simulink model "ampelkreuzungV1.1"  (R2024b)
settings: Solver=FixedStepAuto  StartTime=0.0  StopTime=300  FixedStep=1  RelTol=1e-3
model workspace (MATLAB code in the model file):
  | function [autos_l1, autos_rg1, autos_2l, autos_2rg, autos_3l, autos_3rg, autos_4, fehler] = generateCars(Auslastung)
  |     if (auslastung == 1)
  |         autos_l1 = round(randn());
  |         autos_rg1 = round(randn());
  |         autos_2l = round(randn());
  |         autos_2rg = round(randn());
  |         autos_3l = round(randn());
  |         autos_3rg = round(randn());
  |         autos_4 = round(randn());
  |     else
  |         fehler = 1;
  |     end
  | 
  |     if (auslastung == 2)
  |         autos_l1 = round(randn());
  |         autos_rg1 = round(4 + 2 * randn());
  |         autos_2l = round(1 + randn());
  |         autos_2rg = round(4 + 2 * randn());
  |         autos_3l = round(randn());
  |         autos_3rg = round(2 + randn());
  |         autos_4 = round(1 + randn());
  |     else
  |         fehler = 1;
  |     end
  | 
  |     if (auslastung == 3)
  |         autos_l1 = round(1.5 + randn());
  |         autos_rg1 = round(7 + 2 * randn());
  |         autos_2l = round(2 + randn());
  |         autos_2rg = round(7 + 2 * randn());
  |         autos_3l = round(2 * randn());
  |         autos_3rg = round(3 + randn());
  |         autos_4 = round(2 + randn());
  |     else
  |         fehler = 1;
  |     end
  | 
  |     if (auslastung == 4)
  |         autos_l1 = round(2.5 + randn());
  |         autos_rg1 = round(13 + 3 * randn());
  |         autos_2l = round(5 + randn());
  |         autos_2rg = round(13 + 3 * randn());
  |         autos_3l = round(2 + randn());
  |         autos_3rg = round(2 + randn());
  |         autos_4 = round(5 + randn());
  |     else
  |         fehler = 1;
  |     end
  | end
settings Model: Creator=richa  LastModifiedBy=richa

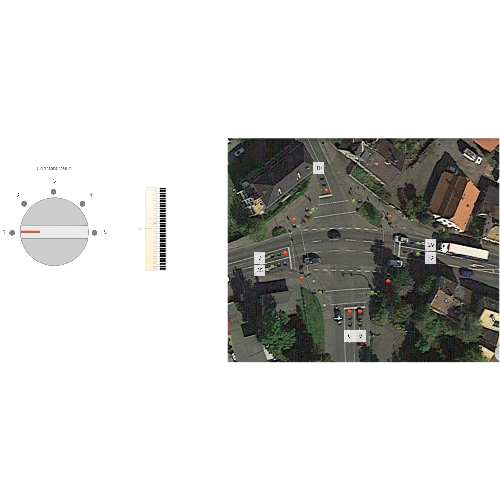
[thumbnail: Simulink's stored preview of the top-level diagram]
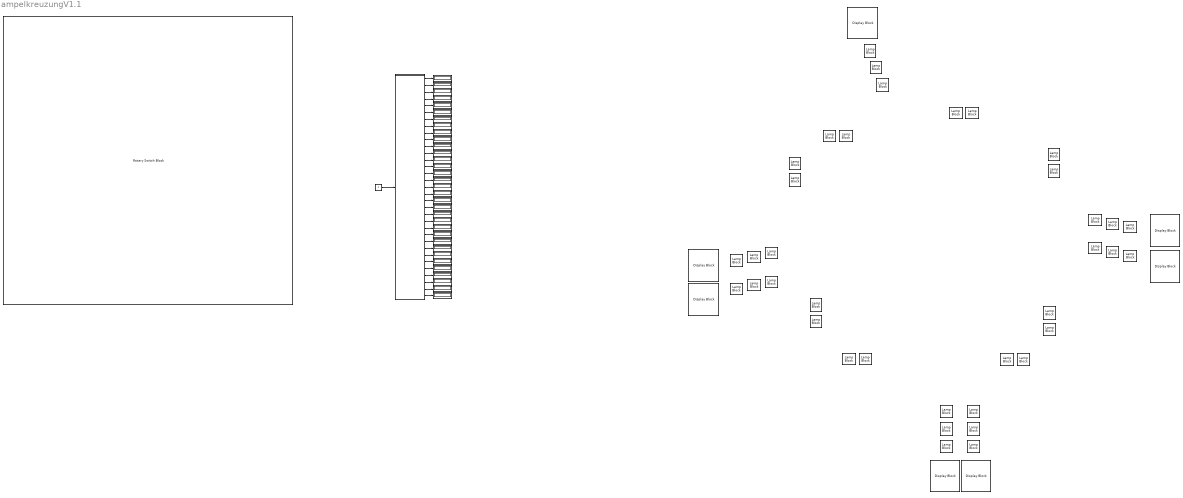
== system ampelkreuzungV1.1 ==
  Chart : Stateflow chart  TreatAsAtomicUnit=on
  Constant : Constant
  Display{,1..26,28..33} (33 alike) : Display
  Display{27,34..37,39..40} (7 alike) : DisplayBlock  LabelPosition=Hide  Transparency=1  Layout=Fill available space
  Lamp{,1..36} (37 alike) : LampBlock  LabelPosition=Hide
  Rotary Switch : RotarySwitchBlock
      settings: Values={{'1', '2', '3', '4', '5'}, [1 2 3 4 5]}
  wires:
  Chart/1(rot1_l) -> Display/1
  Chart/2(gelb1_l) -> Display1/1
  Chart/3(gruen1_l) -> Display2/1
  Chart/4(rot1_rg) -> Display3/1
  Chart/5(gelb1_rg) -> Display4/1
  Chart/6(gruen1_rg) -> Display5/1
  Chart/7(rot2) -> Display6/1
  Chart/8(gelb2) -> Display7/1
  Chart/9(gruen2) -> Display8/1
  Chart/10(rot3_l) -> Display9/1
  Chart/11(gelb3_l) -> Display10/1
  Chart/12(gruen3_l) -> Display11/1
  Chart/13(rot3_rg) -> Display12/1
  Chart/14(gelb3_rg) -> Display13/1
  Chart/15(gruen3_rg) -> Display14/1
  Chart/16(rot4) -> Display15/1
  Chart/17(gelb4) -> Display16/1
  Chart/18(gruen4) -> Display17/1
  Chart/19(rot5) -> Display18/1
  Chart/20(gruen5) -> Display19/1
  Chart/21(rot6) -> Display20/1
  Chart/22(gruen6) -> Display21/1
  Chart/23(rot7) -> Display22/1
  Chart/24(gruen7) -> Display23/1
  Chart/25(rot8) -> Display24/1
  Chart/26(gruen8) -> Display25/1
  Chart/27(autos_1l) -> Display26/1
  Chart/28(autos_1rg) -> Display28/1
  Chart/29(autos_2l) -> Display29/1
  Chart/30(autos_2rg) -> Display30/1
  Chart/31(autos_3l) -> Display31/1
  Chart/32(autos_3rg) -> Display32/1
  Chart/33(autos_4) -> Display33/1
  Constant/1 -> Chart/1(auslastung_eingang)

== stateflow chart ampelkreuzungV1.1/Chart ==
  state Start
    entry:
    rot1_l = 1;
    gelb1_l = 0;
    gruen1_l = 0;
    rot1_rg = 1;
    gelb1_rg = 0;
    gruen1_rg = 0;
    rot2 = 1;
    gelb2 = 0;
    gruen2 = 0;
    rot3_l = 1;
    gelb3_l = 0;
    gruen3_l = 0;
    rot3_rg = 1;
    gelb3_rg = 0;
    gruen3_rg = 0;
    rot4 = 1;
    gelb4 = 0;
    gruen4 = 0;
    rot5 = 1;
    gruen5 = 0;
    rot6 = 1;
    gruen6 = 0;
    rot7 = 1;
    gruen7 = 0;
    rot8 = 1;
    gruen8 = 0;
    restliche_autos = [0 0 0 0 0 0 0];
    kapazitaet = [5 + randn(),  20 + 3 * randn(), 30 + 3 * randn(), 5 + 2 * randn(), 8 + 2 * randn(), 20 + 3 * randn(),  25 + 3 * randn(), 5 + randn(), 8 + 2 * randn(), 8 + 2 * randn()];
    %matrix, runden direkt
  state Autozuweisung
    entry:
    autos_1l = autos(1) + restliche_autos(1);
    autos_1rg = autos(2) + restliche_autos(2);
    autos_2l = autos(3) + restliche_autos(3);
    autos_2rg = autos(4) + restliche_autos(4);
    autos_3l = autos(5) + restliche_autos(5);
    autos_3rg = autos(6) + restliche_autos(6);
    autos_4 = autos(7) + restliche_autos(7);
  state l1_rg1_rotgelb
    entry:
    gelb1_l = 1;
    gelb1_rg = 1;
  state rg1_ampel2_rotgelb
    entry:
    gelb1_rg = 1;
    gelb2 = 1;
  state l1_rg1_gruen
    entry:
    rot1_l = 0;
    gelb1_l = 0;
    gruen1_l = 1;
    rot1_rg = 0;
    gelb1_rg = 0;
    gruen1_rg = 1;
    rot7 = 0;
    gruen7 = 1;
  state rg1_ampel2_gruen
    entry:
    rot1_rg = 0;
    gelb1_rg = 0;
    gruen1_rg = 1;
    rot2 = 0;
    gelb2 = 0;
    gruen2 = 1;
    rot7 = 0;
    gruen7 = 1;
    rot8 = 0;
    gruen8 = 1;
  state l1_gelb
    entry:
    gelb1_l = 1;
    gruen1_l = 0;
  state l1_rot
    entry:
    rot1_l = 1;
    gelb1_l = 0;
  state neu_autos1l
    entry:
    autos_1l = restliche_autos(1)
  state ampel2_rotgelb
    entry:
    gelb2 = 1;
  state ampel2_fuss8_gruen
    rot2 = 0;
    gelb2 = 0;
    gruen2 = 1;
    rot8 = 0;
    gruen8 = 1;
  state Fuss7_rot
    entry:
    rot7 = 1;
    gruen7 = 0;
  state rg1_gelb
    entry:
    gelb1_rg = 1;
    gruen1_rg = 0;
  state rg1_rot
    entry:
    gelb1_rg = 0;
    rot1_rg = 1;
  state neu_autos1rg
    entry:
    autos_1rg = restliche_autos(2)
  state rg1_rot2
    entry:
    gelb1_rg = 0;
    rot1_rg = 1;
  state rg1_rot1
    entry:
    gelb1_rg = 0;
    rot1_rg = 1;
  state fuss8_rot
    entry:
    rot8 = 1;
    gruen8 = 0;
  state ampel2_gelb
    entry:
    gelb2 = 1;
    gruen2 = 0;
  state ampel2_rot
    rot2 = 1;
    gelb2 = 0;
  state neu_autos2l
    entry:
    autos_2l = restliche_autos(3)
  state neu_autos2rg
    entry:
    autos_2rg = restliche_autos(4)
  state rg3_rotgelb
    entry:
    gelb3_rg = 1;
  state l3_rotgelb_rg3_fuss6_gruen
    entry:
    gelb3_l = 1;
    rot3_rg = 0;
    gelb3_rg = 0;
    gruen3_rg = 1;
    rot6 = 0;
    gruen6 = 1;
  state rg3_fuss6_gruen
    entry:
    rot3_rg = 0;
    gelb3_rg = 0;
    gruen3_rg = 1;
    rot6 = 0;
    gruen6 = 1;
  state l3_gruen
    entry:
    rot3_l = 0;
    gelb3_l = 0;
    gruen3_l = 1;
  state l3_gelb
    entry:
    gelb3_l = 1;
    gruen3_l = 0;
  state ampel4_rotgelb
    entry:
    gelb4 = 1;
  state l3_fuss6_rot
    entry:
    rot3_l = 1;
    gelb3_l = 0;
    rot6 = 1;
    gruen6 = 0;
  state ampel4_fuss5_gruen
    entry:
    rot4 = 0;
    gelb4 = 0;
    gruen4 = 1;
    rot5 = 0;
    gruen5 = 1;
  state neu_autos3l
    entry:
    autos_3l = restliche_autos(5)
  state fuss6_rot
    entry:
    rot6 = 1;
    gruen6 = 0;
  state rg3_gelb1
    entry:
    gelb3_rg = 1;
    gruen3_rg = 0;
  state rg3_gelb
    entry:
    gelb3_rg = 1;
    gruen3_rg = 0;
  state rg3_rot_ampel4_rotgelb
    entry:
    rot3_rg = 1;
    gelb3_rg = 0;
    gelb4 = 1;
  state rg3_fuss5_rot
    entry:
    rot3_rg = 1;
    gelb3_rg = 0;
    rot5 = 1;
    gruen5 = 0;
  state neu_autos3rg
    entry:
    autos_3rg = restliche_autos(6)
  state neu_autos3rg1
    entry:
    autos_3rg = restliche_autos(6)
  state ampel4_fuss5_gruen1
    entry:
    rot4 = 0;
    gelb4 = 0;
    gruen4 = 1;
    rot5 = 0;
    gruen5 = 1;
  state fuss5_rot
    entry:
    rot5 = 1;
    gruen5 = 0;
  state ampel4_gelb
    entry:
    gelb4 = 1;
    gruen4 = 0;
  state ampel4_rot
    entry:
    rot4 = 1;
    gelb4 = 0;
  state neu_autos4
    entry:
    autos_4 = restliche_autos(7)
  (default) -> Start
  Start -> (junction 248)
  (junction 181) -> (junction 248)
  (junction 179) -> (junction 181)
  (junction 248) -> Autozuweisung : {autos = generiereAutos(auslastung_eingang)}
  Autozuweisung -> (junction 250)
  (junction 250) -> (junction 15) : after(1,sec)
      |
      | %Linksabbieger1
  (junction 15) -> (junction 69) [order 1] : [autos_1l == 0]
  (junction 15) -> (junction 17) [order 2]
  (junction 69) -> rg1_ampel2_rotgelb
  (junction 17) -> (junction 18) [order 1] : [autos_1l >= 0]
  (junction 17) -> (junction 19) [order 2]
  (junction 18) -> l1_rg1_rotgelb
  l1_rg1_rotgelb -> l1_rg1_gruen : after(1,sec)
  rg1_ampel2_rotgelb -> rg1_ampel2_gruen : after(1,sec)
  l1_rg1_gruen -> l1_gelb : after(7,sec)
  l1_gelb -> l1_rot : after(3,sec)
  rg1_ampel2_gruen -> (junction 71)
  l1_rot -> neu_autos1l : {restliche_autos(1) = subtrahiereAutos(autos_1l, kapazitaet(1))}
  neu_autos1l -> ampel2_rotgelb : after(3,sec)
  ampel2_rotgelb -> ampel2_fuss8_gruen : after(1,sec)
  ampel2_fuss8_gruen -> (junction 20)
  (junction 20) -> (junction 19)
  (junction 71) -> (junction 20)
  (junction 19) -> Fuss7_rot : %Stränge können nicht zusammengeführt werden
      |
      | after(25,sec)
  Fuss7_rot -> rg1_gelb : after(2,sec)
  rg1_gelb -> rg1_rot : after(3,sec)
  rg1_rot -> neu_autos1rg : {restliche_autos(2) = subtrahiereAutos(autos_1rg, kapazitaet(2))}
  neu_autos1rg -> (junction 199) : %Linksabbieger2
  (junction 199) -> (junction 200) [order 1] : [autos_2l == 0]
  (junction 199) -> (junction 201) [order 2]
  (junction 200) -> rg1_rot2
  (junction 201) -> (junction 202) [order 1] : [autos_2l >= 0]
  (junction 201) -> (junction 203) [order 2]
  (junction 202) -> rg1_rot1
  rg1_rot2 -> (junction 205) : %Stränge können nicht zusammengeführt werden, Kapazitäten für Fälle sind unterschiedlich
      |
      | after(7,sec)
  rg1_rot1 -> (junction 204) : after(20,sec)
  (junction 204) -> (junction 203)
  (junction 205) -> (junction 204)
  (junction 203) -> fuss8_rot
  fuss8_rot -> ampel2_gelb : after(2,sec)
  ampel2_gelb -> ampel2_rot : after(3,sec)
  ampel2_rot -> neu_autos2l : {restliche_autos(3) = subtrahiereAutos(autos_2l, kapazitaet(4))}
      | % jeweils 2 unterschiedliche Kapazitäten, Fälle bearbeiten!
  neu_autos2l -> neu_autos2rg : {restliche_autos(4) = subtrahiereAutos(autos_2rg, kapazitaet(6))}
  neu_autos2rg -> rg3_rotgelb : after(1,sec)
  rg3_rotgelb -> (junction 115) : %Linksabbieger3
  (junction 115) -> (junction 116) [order 1] : [autos_3l == 0]
  (junction 115) -> (junction 117) [order 2]
  (junction 116) -> rg3_fuss6_gruen : after(1,sec)
  (junction 117) -> (junction 118) [order 1] : [autos_3l >= 0]
  (junction 117) -> (junction 119) [order 2]
  (junction 118) -> l3_rotgelb_rg3_fuss6_gruen
  l3_rotgelb_rg3_fuss6_gruen -> l3_gruen
  rg3_fuss6_gruen -> ampel4_rotgelb : after(4,sec)
  l3_gruen -> l3_gelb : after(8,sec)
  l3_gelb -> l3_fuss6_rot : after(3,sec)
  ampel4_rotgelb -> ampel4_fuss5_gruen : after(1,sec)
  l3_fuss6_rot -> neu_autos3l : {restliche_autos(5) = subtrahiereAutos(autos_3l, kapazitaet(8))}
  ampel4_fuss5_gruen -> fuss6_rot : after(6,sec)
  neu_autos3l -> rg3_gelb1 : after(2,sec)
  fuss6_rot -> rg3_gelb : after(2,sec)
  rg3_gelb1 -> rg3_rot_ampel4_rotgelb : after(3,sec)
  rg3_gelb -> rg3_fuss5_rot : after(3,sec)
  rg3_rot_ampel4_rotgelb -> neu_autos3rg : {restliche_autos(6) = subtrahiereAutos(autos_3rg, kapazitaet(9))}
  rg3_fuss5_rot -> neu_autos3rg1 : {restliche_autos(6) = subtrahiereAutos(autos_3rg, kapazitaet(9))}
  neu_autos3rg -> ampel4_fuss5_gruen1 : after(1,sec)
  neu_autos3rg1 -> (junction 121)
  ampel4_fuss5_gruen1 -> fuss5_rot : after(11,sec)
  fuss5_rot -> (junction 120)
  (junction 120) -> (junction 119)
  (junction 121) -> (junction 120)
  (junction 119) -> (junction 122)
  (junction 122) -> ampel4_gelb : after(2,sec)
  ampel4_gelb -> ampel4_rot : after(3,sec)
  ampel4_rot -> neu_autos4 : {restliche_autos(7) = subtrahiereAutos(autos_4, kapazitaet(10))}
  neu_autos4 -> (junction 177) : after(4,sec)
  (junction 177) -> (junction 179)
  data: anzahl_autos_pro_spur function_output; auslastung function_input; anzahl_autos_pro_spur function_input; verbleibende_autos function_output; maximale_kapazitaet function_input; rot1_l output; gelb1_l output; gruen1_l output; rot1_rg output; gelb1_rg output; gruen1_rg output; rot2 output; gelb2 output; gruen2 output; rot3_l output; gelb3_l output; gruen3_l output; rot3_rg output; gelb3_rg output; gruen3_rg output; rot4 output; gelb4 output; gruen4 output; rot5 output; gruen5 output; rot6 output; gruen6 output; rot7 output; gruen7 output; rot8 output; gruen8 output; autos_1l output; autos_1rg output; autos_2l output; autos_2rg output; autos_3l output; autos_3rg output; autos_4 output; autos local; auslastung_eingang input; restliche_autos local; kapazitaet local
  function anzahl_autos_pro_spur = generiereAutos(auslastung):
    | function anzahl_autos_pro_spur = generiereAutos(auslastung)
    | 
    |     if (auslastung == 1)
    |         autos_1l = round(0.5 * randn());
    |         autos_1rg = round(0.5 * randn());
    |         autos_2l = round(0.5 * randn());
    |         autos_2rg = round(0.5 * randn());
    |         autos_3l = round(0.5 * randn());
    |         autos_3rg = round(0.5 * randn());
    |         autos_4 = round(0.5 * randn());
    |     elseif (auslastung == 2)
    |         autos_1l = round(randn());
    |         autos_1rg = round(4 + 2 * randn());
    |         autos_2l = round(1 + randn());
    |         autos_2rg = round(4 + 2 * randn());
    |         autos_3l = round(randn());
    |         autos_3rg = round(2 + randn());
    |         autos_4 = round(1 + randn());
    |     elseif (auslastung == 3)
    |         autos_1l = round(1.5 + randn());
    |         autos_1rg = round(7 + 2 * randn());
    |         autos_2l = round(2 + randn());
    |         autos_2rg = round(7 + 2 * randn());
    |         autos_3l = round(2 * randn());
    |         autos_3rg = round(3 + randn());
    |         autos_4 = round(2 + randn());
    |     elseif (auslastung == 4)
    |         autos_1l = round(2.5 + randn());
    |         autos_1rg = round(13 + 3 * randn());
    |         autos_2l = round(5 + randn());
    |         autos_2rg = round(13 + 3 * randn());
    |         autos_3l = round(2 + randn());
    |         autos_3rg = round(5 + randn());
    |         autos_4 = round(5 + randn());
    |     elseif (auslastung == 5)
    |         autos_1l = round(3.5 + randn());
    |         autos_1rg = round(20 + 5 * randn());
    |         autos_2l = round(7 + 2* randn());
    |         autos_2rg = round(20 + 5 * randn());
    |         autos_3l = round(5 + 2 * randn());
    |         autos_3rg = round(8 + 2 * randn());
    |         autos_4 = round(8 + 2 * randn());
    |     else
    |         autos_1l = 0;
    |         autos_1rg = 0;
    |         autos_2l = 0;
    |         autos_2rg = 0;
    |         autos_3l = 0;
    |         autos_3rg = 0;
    |         autos_4 = 0;
    |     end
    | 
    |     anzahl_autos_pro_spur = [autos_1l, autos_1rg, autos_2l, autos_2rg, autos_3l, autos_3rg, autos_4];
    | 
    |     for i = 1:(length(anzahl_autos_pro_spur))
    |         if anzahl_autos_pro_spur(i) < 0
    |             anzahl_autos_pro_spur(i) = 0;
    |         end
    |     end
    | end
  function verbleibende_autos = subtrahiereAutos(anzahl_autos_pro_spur, maximale_kapazitaet):
    | function verbleibende_autos = subtrahiereAutos(anzahl_autos_pro_spur, maximale_kapazitaet)
    |     verbleibende_autos = round(anzahl_autos_pro_spur - maximale_kapazitaet);
    |     if (verbleibende_autos < 0)
    |         verbleibende_autos = 0;
    |     end
    | end
